simulink model "ScpAp_VechilestateEstimation_L2p"  (R2025b)
settings: Solver=FixedStepDiscrete  StartTime=0.0  StopTime=10.0  FixedStep=0.01  RelTol=1e-3
model workspace (MAT data in the model file):
  Accel_Diff_Th = Simulink.Parameter
  Accel_Diff_Th.Value = 1
  Accel_Diff_Th.Complexity = 'real'
  Accel_Diff_Th.Dimensions = [1 1]
  Accel_Diff_Th.DataType = 'auto'
  DT = Simulink.Parameter
  DT.Value = 0.01
  DT.Complexity = 'real'
  DT.Dimensions = [1 1]
  DT.DataType = 'auto'
  Speed_Diff_Th = Simulink.Parameter
  Speed_Diff_Th.Value = 4
  Speed_Diff_Th.Complexity = 'real'
  Speed_Diff_Th.Dimensions = [1 1]
  Speed_Diff_Th.DataType = 'auto'
  W1 = Simulink.Parameter
  W1.Value = 0.3
  W1.Complexity = 'real'
  W1.Dimensions = [1 1]
  W1.DataType = 'auto'
  W2 = Simulink.Parameter
  W2.Value = 0.7
  W2.Complexity = 'real'
  W2.Dimensions = [1 1]
  W2.DataType = 'auto'
  Wheel_Diff_Th = Simulink.Parameter
  Wheel_Diff_Th.Value = 5
  Wheel_Diff_Th.Complexity = 'real'
  Wheel_Diff_Th.Dimensions = [1 1]
  Wheel_Diff_Th.DataType = 'auto'
undefined symbols (not defined in the file): w_accel1, w_accel2, WhlSpd_Max, WhlSpd_Min
settings Model: DataDictionary=EgasPOC.sldd  Creator=IAST283  LastModifiedBy=IAST283
settings DataIOCC: SaveFormat=StructureWithTime
settings OptimizationCC: DefaultParameterBehavior=Inlined  EnhancedBackFolding=on  PassReuseOutputArgsAs=Individual arguments  ZeroExternalMemoryAtStartup=off  ZeroInternalMemoryAtStartup=off  OptimizeBlockOrder=speed  DifferentSizesBufferReuse=on  OptimizationCustomize=off  EfficientTunableParamExpr=on
settings DebuggingCC: ParameterTunabilityLossMsg=error
settings SFSimCC: MATLABDynamicMemAlloc=off
settings RTWCC: SystemTargetFile=autosar.tlc  GenCodeOnly=on  TemplateMakefile=ert_default_tmf  DataTypeReplacement=CDataTypesFixedWidth  Description=AUTOSAR
settings CodeAppCC: ForceParamTrailComments=on  IgnoreCustomStorageClasses=off  OperatorAnnotations=on  SimulinkDataObjDesc=on  SFDataObjDesc=on  InsertBlockDesc=on
settings STFCustomTargetCC: SystemTargetFile=autosar.tlc  TargetLangStandard=C99 (ISO)  MultiwordLength=256.0  ParMdlRefBuildCompliant=on  CompOptLevelCompliant=on  ConcurrentExecutionCompliant=off  IncludeMdlTerminateFcn=off  CombineOutputUpdateFcns=on  SuppressErrorStatus=on  ERTCustomFileBanners=on  SupportNonFinite=off  SupportComplex=off  SupportContinuousTime=off  SupportNonInlinedSFcns=off  RemoveResetFunc=on  MATLABClassNameForMDSCustomization=Simulink.SoftwareTarget.ERTCustomization  AutosarCompliant=on  GRTInterface=off  UseToolchainInfoCompliant=on  LookupTableObjectStructAxisOrder=2,1,3,4,...  LUTObjectStructOrderEvenSpacing=Size,Table,Breakpoints  AutosarCompilerAbstraction=off  DisableAUTOSARRoutinesHostLibrary=off  AutosarSchemaVersion=R23-11  AutosarMaxShortNameLength=128.0  AutosarMatrixIOAsArray=off
settings ERTTargetCC: ERTCustomFileTemplate=example_file_process.tlc  BooleanTrueId=TRUE  BooleanFalseId=FALSE  TargetLangStandard=C99 (ISO)  ConcurrentExecutionCompliant=off  IncludeMdlTerminateFcn=off  SuppressErrorStatus=on  SupportNonFinite=off  SupportComplex=off  ModelStepFunctionPrototypeControlCompliant=off  CPPClassGenCompliant=off  AutosarCompliant=on  LookupTableObjectStructAxisOrder=2,1,3,4,...  LUTObjectStructOrderEvenSpacing=Size,Table,Breakpoints

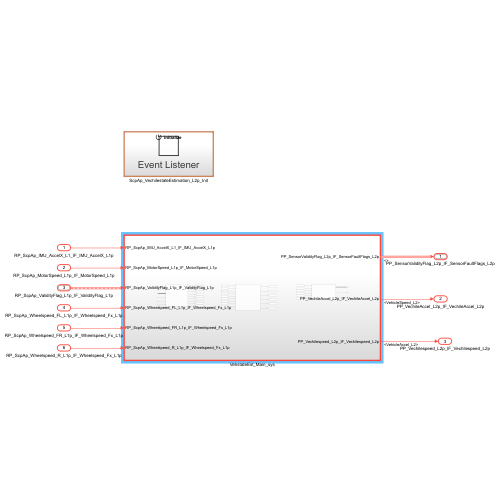
[thumbnail: Simulink's stored preview of the top-level diagram]
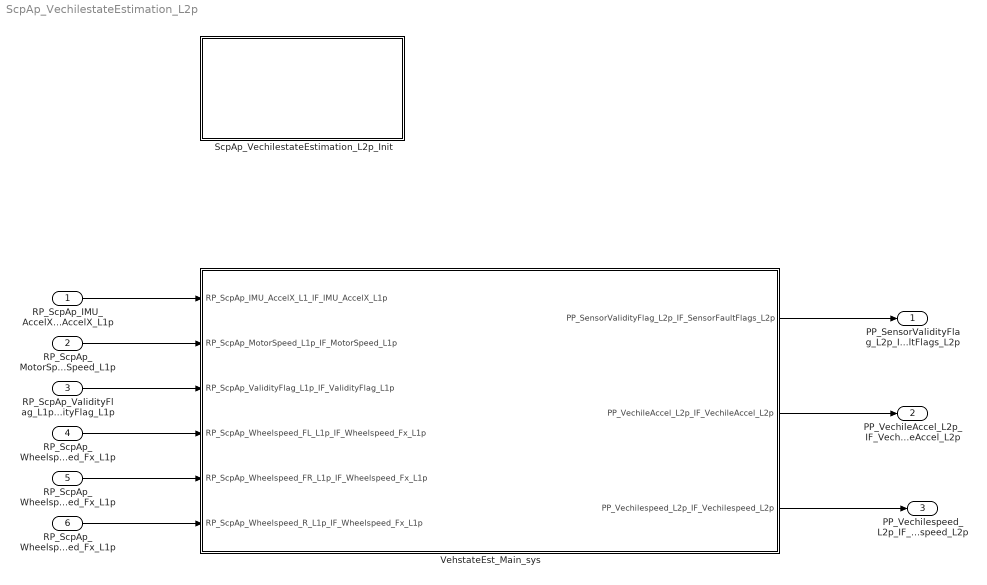
== system ScpAp_VechilestateEstimation_L2p ==
  RP_ScpAp_IMU_AccelX_L1_IF_IMU_AccelX_L1p : Inport  OutDataTypeStr=single  PortDimensions=1
  RP_ScpAp_MotorSpeed_L1p_IF_MotorSpeed_L1p : Inport  Port=2  OutDataTypeStr=uint8  PortDimensions=1
  RP_ScpAp_ValidityFlag_L1p_IF_ValidityFlag_L1p : Inport  Port=3  OutDataTypeStr=Bus: IF_ValidityFlag_L1p_IDT  PortDimensions=1  BusOutputAsStruct=on
  RP_ScpAp_Wheelspeed_FL_L1p_IF_Wheelspeed_Fx_L1p : Inport  Port=4  OutDataTypeStr=uint16  PortDimensions=1
  RP_ScpAp_Wheelspeed_FR_L1p_IF_Wheelspeed_Fx_L1p : Inport  Port=5  OutDataTypeStr=uint16  PortDimensions=1
  RP_ScpAp_Wheelspeed_R_L1p_IF_Wheelspeed_Fx_L1p : Inport  Port=6  OutDataTypeStr=uint16  PortDimensions=1
  ScpAp_VechilestateEstimation_L2p_Init : Subsystem
  VehstateEst_Main_sys : Subsystem  TreatAsAtomicUnit=on  SystemSampleTime=0.01
  PP_SensorValidityFlag_L2p_IF_SensorFaultFlags_L2p : Outport  OutDataTypeStr=Bus: IF_SensorFaultFlgs_L2p_IDT  PortDimensions=1  BusOutputAsStruct=on
  PP_VechileAccel_L2p_IF_VechileAccel_L2p : Outport  Port=2  OutDataTypeStr=int16  PortDimensions=1
  PP_Vechilespeed_L2p_IF_Vechilespeed_L2p : Outport  Port=3  OutDataTypeStr=uint16  PortDimensions=1
  wires:
  VehstateEst_Main_sys/1(PP_SensorValidityFlag_L2p_IF_SensorFaultFlags_L2p) -> PP_SensorValidityFlag_L2p_IF_SensorFaultFlags_L2p/1
  VehstateEst_Main_sys/2(PP_VechileAccel_L2p_IF_VechileAccel_L2p) -> PP_VechileAccel_L2p_IF_VechileAccel_L2p/1
  VehstateEst_Main_sys/3(PP_Vechilespeed_L2p_IF_Vechilespeed_L2p) -> PP_Vechilespeed_L2p_IF_Vechilespeed_L2p/1
  RP_ScpAp_IMU_AccelX_L1_IF_IMU_AccelX_L1p/1 -> VehstateEst_Main_sys/1(RP_ScpAp_IMU_AccelX_L1_IF_IMU_AccelX_L1p)
  RP_ScpAp_MotorSpeed_L1p_IF_MotorSpeed_L1p/1 -> VehstateEst_Main_sys/2(RP_ScpAp_MotorSpeed_L1p_IF_MotorSpeed_L1p)
  RP_ScpAp_ValidityFlag_L1p_IF_ValidityFlag_L1p/1 -> VehstateEst_Main_sys/3(RP_ScpAp_ValidityFlag_L1p_IF_ValidityFlag_L1p)
  RP_ScpAp_Wheelspeed_FL_L1p_IF_Wheelspeed_Fx_L1p/1 -> VehstateEst_Main_sys/4(RP_ScpAp_Wheelspeed_FL_L1p_IF_Wheelspeed_Fx_L1p)
  RP_ScpAp_Wheelspeed_FR_L1p_IF_Wheelspeed_Fx_L1p/1 -> VehstateEst_Main_sys/5(RP_ScpAp_Wheelspeed_FR_L1p_IF_Wheelspeed_Fx_L1p)
  RP_ScpAp_Wheelspeed_R_L1p_IF_Wheelspeed_Fx_L1p/1 -> VehstateEst_Main_sys/6(RP_ScpAp_Wheelspeed_R_L1p_IF_Wheelspeed_Fx_L1p)

== system ScpAp_VechilestateEstimation_L2p/ScpAp_VechilestateEstimation_L2p_Init ==
  Event Listener : EventListener  EventName=reset

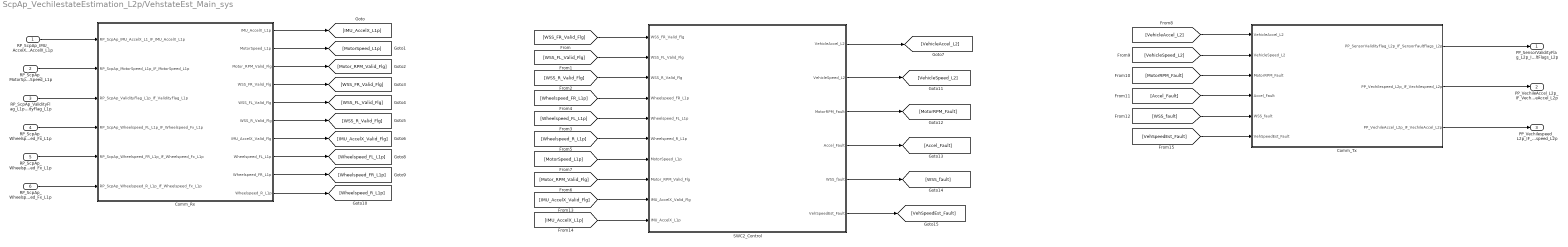
== system ScpAp_VechilestateEstimation_L2p/VehstateEst_Main_sys ==
  RP_ScpAp_IMU_AccelX_L1_IF_IMU_AccelX_L1p : Inport  OutDataTypeStr=single  PortDimensions=1
  RP_ScpAp_MotorSpeed_L1p_IF_MotorSpeed_L1p : Inport  Port=2  OutDataTypeStr=uint8  PortDimensions=1
  RP_ScpAp_ValidityFlag_L1p_IF_ValidityFlag_L1p : Inport  Port=3  OutDataTypeStr=Bus: IF_ValidityFlag_L1p_IDT  PortDimensions=1  BusOutputAsStruct=on
  RP_ScpAp_Wheelspeed_FL_L1p_IF_Wheelspeed_Fx_L1p : Inport  Port=4  OutDataTypeStr=uint16  PortDimensions=1
  RP_ScpAp_Wheelspeed_FR_L1p_IF_Wheelspeed_Fx_L1p : Inport  Port=5  OutDataTypeStr=uint16  PortDimensions=1
  RP_ScpAp_Wheelspeed_R_L1p_IF_Wheelspeed_Fx_L1p : Inport  Port=6  OutDataTypeStr=uint16  PortDimensions=1
  Comm_Rx : Subsystem
  Comm_Tx : Subsystem
  SWC2_Control : Subsystem  TreatAsAtomicUnit=on
  PP_SensorValidityFlag_L2p_IF_SensorFaultFlags_L2p : Outport
  PP_VechileAccel_L2p_IF_VechileAccel_L2p : Outport  Port=2
  PP_Vechilespeed_L2p_IF_Vechilespeed_L2p : Outport  Port=3
  wires:
  Comm_Rx/4(WSS_FR_Valid_Flg) -> [WSS_FR_Valid_Flg]
  Comm_Rx/3(Motor_RPM_Valid_Flg) -> [Motor_RPM_Valid_Flg]
  Comm_Rx/2(MotorSpeed_L1p) -> [MotorSpeed_L1p]
  Comm_Rx/8(Wheelspeed_FL_L1p) -> [Wheelspeed_FL_L1p]
  Comm_Rx/10(Wheelspeed_R_L1p) -> [Wheelspeed_R_L1p]
  Comm_Rx/9(Wheelspeed_FR_L1p) -> [Wheelspeed_FR_L1p]
  Comm_Rx/1(IMU_AccelX_L1p) -> [IMU_AccelX_L1p]
  Comm_Rx/7(IMU_AccelX_Valid_Flg) -> [IMU_AccelX_Valid_Flg]
  Comm_Rx/5(WSS_FL_Valid_Flg) -> [WSS_FL_Valid_Flg]
  Comm_Rx/6(WSS_R_Valid_Flg) -> [WSS_R_Valid_Flg]
  RP_ScpAp_IMU_AccelX_L1_IF_IMU_AccelX_L1p/1 -> Comm_Rx/1(RP_ScpAp_IMU_AccelX_L1_IF_IMU_AccelX_L1p)
  RP_ScpAp_MotorSpeed_L1p_IF_MotorSpeed_L1p/1 -> Comm_Rx/2(RP_ScpAp_MotorSpeed_L1p_IF_MotorSpeed_L1p)
  SWC2_Control/1("VehicleAccel_L2 ") -> [VehicleAccel_L2]
  SWC2_Control/3("MotorRPM_Fault ") -> [MotorRPM_Fault]
  [Wheelspeed_R_L1p] -> SWC2_Control/6(Wheelspeed_R_L1p)
  [IMU_AccelX_L1p] -> SWC2_Control/10(IMU_AccelX_L1p)
  SWC2_Control/6(VehSpeedEst_Fault) -> [VehSpeedEst_Fault]
  [MotorSpeed_L1p] -> SWC2_Control/7(MotorSpeed_L1p)
  [WSS_R_Valid_Flg] -> SWC2_Control/3(WSS_R_Valid_Flg)
  [IMU_AccelX_Valid_Flg] -> SWC2_Control/9(IMU_AccelX_Valid_Flg)
  [Wheelspeed_FR_L1p] -> SWC2_Control/4(Wheelspeed_FR_L1p)
  [Motor_RPM_Valid_Flg] -> SWC2_Control/8(Motor_RPM_Valid_Flg)
  [WSS_FR_Valid_Flg] -> SWC2_Control/1(WSS_FR_Valid_Flg)
  SWC2_Control/4(Accel_Fault) -> [Accel_Fault]
  [Wheelspeed_FL_L1p] -> SWC2_Control/5(Wheelspeed_FL_L1p)
  SWC2_Control/2("VehicleSpeed_L2 ") -> [VehicleSpeed_L2]
  [WSS_FL_Valid_Flg] -> SWC2_Control/2(WSS_FL_Valid_Flg)
  SWC2_Control/5("WSS_fault ") -> [WSS_fault]
  [VehicleAccel_L2] -> Comm_Tx/1(VehicleAccel_L2)
  [Accel_Fault] -> Comm_Tx/4(Accel_Fault)
  [MotorRPM_Fault] -> Comm_Tx/3(MotorRPM_Fault)
  [VehSpeedEst_Fault] -> Comm_Tx/6(VehSpeedEst_Fault)
  [WSS_fault] -> Comm_Tx/5(WSS_fault)
  [VehicleSpeed_L2] -> Comm_Tx/2(VehicleSpeed_L2)
  Comm_Tx/3(PP_VechileAccel_L2p_IF_VechileAccel_L2p) -> PP_Vechilespeed_L2p_IF_Vechilespeed_L2p/1
  Comm_Tx/1(PP_SensorValidityFlag_L2p_IF_SensorFaultFlags_L2p) -> PP_SensorValidityFlag_L2p_IF_SensorFaultFlags_L2p/1
  Comm_Tx/2(PP_Vechilespeed_L2p_IF_Vechilespeed_L2p) -> PP_VechileAccel_L2p_IF_VechileAccel_L2p/1
  RP_ScpAp_ValidityFlag_L1p_IF_ValidityFlag_L1p/1 -> Comm_Rx/3(RP_ScpAp_ValidityFlag_L1p_IF_ValidityFlag_L1p)
  RP_ScpAp_Wheelspeed_R_L1p_IF_Wheelspeed_Fx_L1p/1 -> Comm_Rx/6(RP_ScpAp_Wheelspeed_R_L1p_IF_Wheelspeed_Fx_L1p)
  RP_ScpAp_Wheelspeed_FR_L1p_IF_Wheelspeed_Fx_L1p/1 -> Comm_Rx/5(RP_ScpAp_Wheelspeed_FR_L1p_IF_Wheelspeed_Fx_L1p)
  RP_ScpAp_Wheelspeed_FL_L1p_IF_Wheelspeed_Fx_L1p/1 -> Comm_Rx/4(RP_ScpAp_Wheelspeed_FL_L1p_IF_Wheelspeed_Fx_L1p)

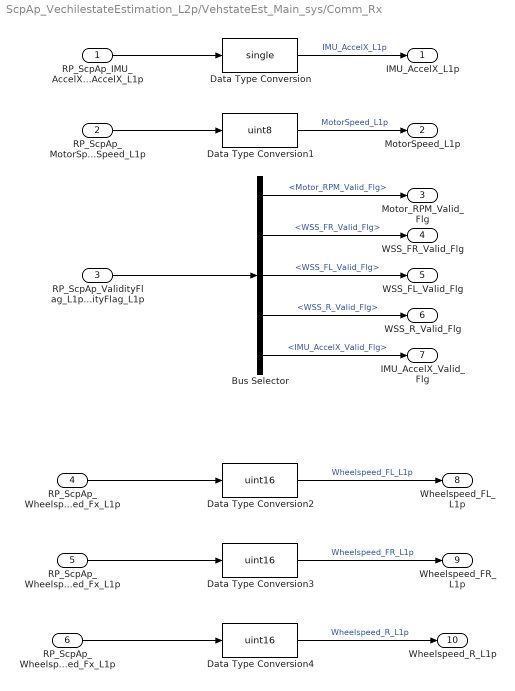
== system ScpAp_VechilestateEstimation_L2p/VehstateEst_Main_sys/Comm_Rx ==
  RP_ScpAp_IMU_AccelX_L1_IF_IMU_AccelX_L1p : Inport  OutDataTypeStr=single
  RP_ScpAp_MotorSpeed_L1p_IF_MotorSpeed_L1p : Inport  Port=2
  RP_ScpAp_ValidityFlag_L1p_IF_ValidityFlag_L1p : Inport  Port=3
  RP_ScpAp_Wheelspeed_FL_L1p_IF_Wheelspeed_Fx_L1p : Inport  Port=4
  RP_ScpAp_Wheelspeed_FR_L1p_IF_Wheelspeed_Fx_L1p : Inport  Port=5
  RP_ScpAp_Wheelspeed_R_L1p_IF_Wheelspeed_Fx_L1p : Inport  Port=6
  Bus Selector : BusSelector  OutputSignals=Motor_RPM_Valid_Flg,WSS_FR_Valid_Flg,WSS_FL_Valid_Flg,WSS_R_Valid_Flg,IMU_AccelX_Valid_Flg
  Data Type Conversion : DataTypeConversion  OutDataTypeStr=single  SaturateOnIntegerOverflow=off  RndMeth=Floor
  Data Type Conversion1 : DataTypeConversion  OutDataTypeStr=uint8  SaturateOnIntegerOverflow=off  RndMeth=Floor
  Data Type Conversion2 : DataTypeConversion  OutDataTypeStr=uint16  SaturateOnIntegerOverflow=off  RndMeth=Floor
  Data Type Conversion3 : DataTypeConversion  OutDataTypeStr=uint16  SaturateOnIntegerOverflow=off  RndMeth=Floor
  Data Type Conversion4 : DataTypeConversion  OutDataTypeStr=uint16  SaturateOnIntegerOverflow=off  RndMeth=Floor
  IMU_AccelX_L1p : Outport  OutDataTypeStr=single
  MotorSpeed_L1p : Outport  Port=2
  Motor_RPM_Valid_Flg : Outport  Port=3
  WSS_FR_Valid_Flg : Outport  Port=4
  WSS_FL_Valid_Flg : Outport  Port=5
  WSS_R_Valid_Flg : Outport  Port=6
  IMU_AccelX_Valid_Flg : Outport  Port=7
  Wheelspeed_FL_L1p : Outport  Port=8
  Wheelspeed_FR_L1p : Outport  Port=9
  Wheelspeed_R_L1p : Outport  Port=10
  wires:
  RP_ScpAp_IMU_AccelX_L1_IF_IMU_AccelX_L1p/1 -> Data Type Conversion/1
  RP_ScpAp_MotorSpeed_L1p_IF_MotorSpeed_L1p/1 -> Data Type Conversion1/1
  RP_ScpAp_ValidityFlag_L1p_IF_ValidityFlag_L1p/1 -> Bus Selector/1
  Bus Selector/1 -> Motor_RPM_Valid_Flg/1  "<Motor_RPM_Valid_Flg>"
  Bus Selector/2 -> WSS_FR_Valid_Flg/1  "<WSS_FR_Valid_Flg>"
  Bus Selector/3 -> WSS_FL_Valid_Flg/1  "<WSS_FL_Valid_Flg>"
  Bus Selector/4 -> WSS_R_Valid_Flg/1  "<WSS_R_Valid_Flg>"
  Bus Selector/5 -> IMU_AccelX_Valid_Flg/1  "<IMU_AccelX_Valid_Flg>"
  RP_ScpAp_Wheelspeed_FL_L1p_IF_Wheelspeed_Fx_L1p/1 -> Data Type Conversion2/1
  RP_ScpAp_Wheelspeed_FR_L1p_IF_Wheelspeed_Fx_L1p/1 -> Data Type Conversion3/1
  RP_ScpAp_Wheelspeed_R_L1p_IF_Wheelspeed_Fx_L1p/1 -> Data Type Conversion4/1
  Data Type Conversion/1 -> IMU_AccelX_L1p/1  "IMU_AccelX_L1p"
  Data Type Conversion1/1 -> MotorSpeed_L1p/1  "MotorSpeed_L1p"
  Data Type Conversion2/1 -> Wheelspeed_FL_L1p/1  "Wheelspeed_FL_L1p"
  Data Type Conversion3/1 -> Wheelspeed_FR_L1p/1  "Wheelspeed_FR_L1p"
  Data Type Conversion4/1 -> Wheelspeed_R_L1p/1  "Wheelspeed_R_L1p"

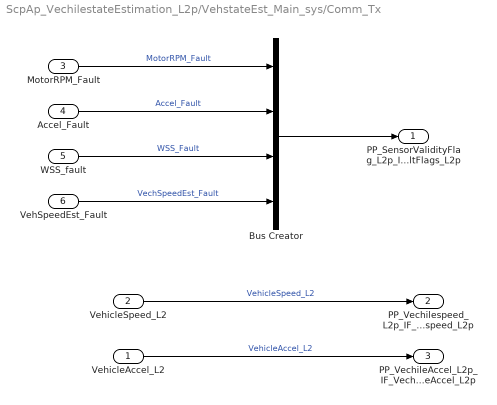
== system ScpAp_VechilestateEstimation_L2p/VehstateEst_Main_sys/Comm_Tx ==
  VehicleAccel_L2 : Inport
  VehicleSpeed_L2 : Inport  Port=2
  MotorRPM_Fault : Inport  Port=3
  Accel_Fault : Inport  Port=4
  WSS_fault : Inport  Port=5
  VehSpeedEst_Fault : Inport  Port=6
  Bus Creator : BusCreator  Inputs=4
  PP_SensorValidityFlag_L2p_IF_SensorFaultFlags_L2p : Outport
  PP_Vechilespeed_L2p_IF_Vechilespeed_L2p : Outport  Port=2
  PP_VechileAccel_L2p_IF_VechileAccel_L2p : Outport  Port=3
  wires:
  MotorRPM_Fault/1 -> Bus Creator/1  "MotorRPM_Fault"
  WSS_fault/1 -> Bus Creator/3  "WSS_Fault"
  Accel_Fault/1 -> Bus Creator/2  "Accel_Fault"
  VehSpeedEst_Fault/1 -> Bus Creator/4  "VechSpeedEst_Fault"
  VehicleAccel_L2/1 -> PP_VechileAccel_L2p_IF_VechileAccel_L2p/1  "VehicleAccel_L2"
  VehicleSpeed_L2/1 -> PP_Vechilespeed_L2p_IF_Vechilespeed_L2p/1  "VehicleSpeed_L2"
  Bus Creator/1 -> PP_SensorValidityFlag_L2p_IF_SensorFaultFlags_L2p/1

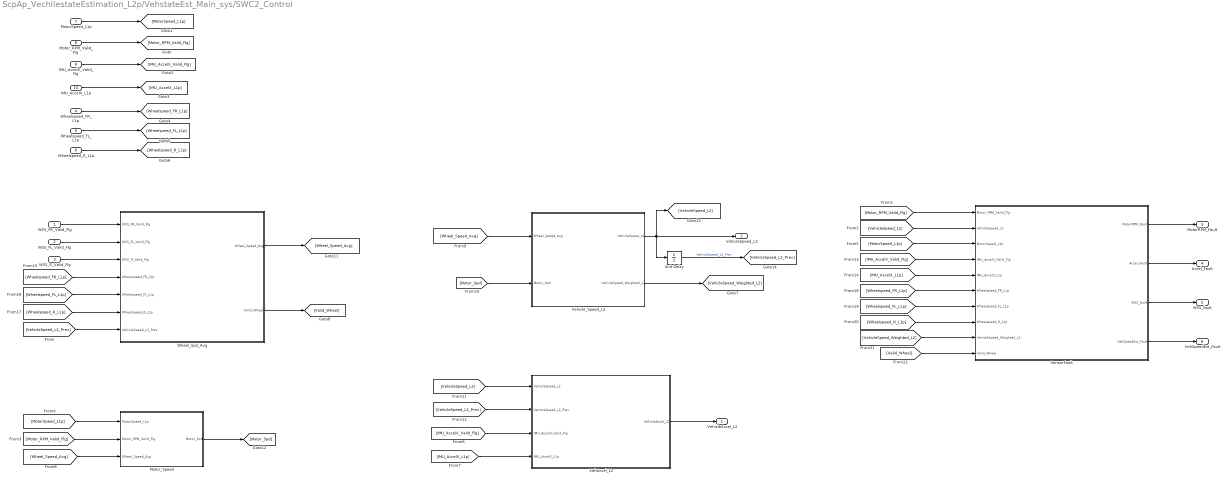
== system ScpAp_VechilestateEstimation_L2p/VehstateEst_Main_sys/SWC2_Control ==
  WSS_FR_Valid_Flg : Inport
  WSS_FL_Valid_Flg : Inport  Port=2
  WSS_R_Valid_Flg : Inport  Port=3
  Wheelspeed_FR_L1p : Inport  Port=4
  Wheelspeed_FL_L1p : Inport  Port=5
  Wheelspeed_R_L1p : Inport  Port=6
  MotorSpeed_L1p : Inport  Port=7
  Motor_RPM_Valid_Flg : Inport  Port=8
  IMU_AccelX_Valid_Flg : Inport  Port=9
  IMU_AccelX_L1p : Inport  Port=10
  Motor_Speed : Subsystem  TreatAsAtomicUnit=on
  SensorFault : Subsystem  TreatAsAtomicUnit=on
  Unit Delay : UnitDelay  SampleTime=-1  HasFrameUpgradeWarning=on
  VehAccel_L2 : Subsystem  TreatAsAtomicUnit=on
  Vehicle_Speed_L2 : Subsystem  TreatAsAtomicUnit=on
  Wheel_Spd_Avg : Subsystem  TreatAsAtomicUnit=on
  "VehicleAccel_L2 " : Outport
  "VehicleSpeed_L2 " : Outport  Port=2
  "MotorRPM_Fault " : Outport  Port=3
  Accel_Fault : Outport  Port=4
  "WSS_fault " : Outport  Port=5
  VehSpeedEst_Fault : Outport  Port=6
  wires:
  [Motor_Spd] -> Vehicle_Speed_L2/2(Motor_Spd)
  Motor_Speed/1(Motor_Spd) -> [Motor_Spd]
  Wheel_Spd_Avg/1(Wheel_Speed_Avg) -> [Wheel_Speed_Avg]
  [Wheel_Speed_Avg] -> Motor_Speed/3(Wheel_Speed_Avg)
  [Wheel_Speed_Avg] -> Vehicle_Speed_L2/1(Wheel_Speed_Avg)
  Unit Delay/1 -> [VehicleSpeed_L2_Prev]  "VehicleSpeed_L2_Prev"
  [VehicleSpeed_L2] -> VehAccel_L2/1(VehicleSpeed_L2)
  [VehicleSpeed_L2_Prev] -> VehAccel_L2/2(VehicleSpeed_L2_Prev)
  WSS_FR_Valid_Flg/1 -> Wheel_Spd_Avg/1(WSS_FR_Valid_Flg)
  WSS_R_Valid_Flg/1 -> Wheel_Spd_Avg/3(WSS_R_Valid_Flg)
  WSS_FL_Valid_Flg/1 -> Wheel_Spd_Avg/2(WSS_FL_Valid_Flg)
  VehAccel_L2/1("VehicleAccel_L2 ") -> "VehicleAccel_L2 "/1
  [VehicleSpeed_L2_Prev] -> Wheel_Spd_Avg/7(VehicleSpeed_L2_Prev)
  Motor_RPM_Valid_Flg/1 -> [Motor_RPM_Valid_Flg]
  [Motor_RPM_Valid_Flg] -> Motor_Speed/2(Motor_RPM_Valid_Flg)
  [MotorSpeed_L1p] -> Motor_Speed/1(MotorSpeed_L1p)
  [Motor_RPM_Valid_Flg] -> SensorFault/1(Motor_RPM_Valid_Flg)
  [VehicleSpeed_L2] -> SensorFault/2(VehicleSpeed_L2)
  [MotorSpeed_L1p] -> SensorFault/3(MotorSpeed_L1p)
  IMU_AccelX_Valid_Flg/1 -> [IMU_AccelX_Valid_Flg]
  IMU_AccelX_L1p/1 -> [IMU_AccelX_L1p]
  [IMU_AccelX_Valid_Flg] -> VehAccel_L2/3(IMU_AccelX_Valid_Flg)
  [IMU_AccelX_L1p] -> VehAccel_L2/4(IMU_AccelX_L1p)
  [IMU_AccelX_Valid_Flg] -> SensorFault/4(IMU_AccelX_Valid_Flg)
  [IMU_AccelX_L1p] -> SensorFault/5(IMU_AccelX_L1p)
  Wheelspeed_FR_L1p/1 -> [Wheelspeed_FR_L1p]
  Wheelspeed_FL_L1p/1 -> [Wheelspeed_FL_L1p]
  Wheelspeed_R_L1p/1 -> [Wheelspeed_R_L1p]
  [Wheelspeed_FR_L1p] -> Wheel_Spd_Avg/4(Wheelspeed_FR_L1p)
  [Wheelspeed_FL_L1p] -> Wheel_Spd_Avg/5(Wheelspeed_FL_L1p)
  [Wheelspeed_R_L1p] -> Wheel_Spd_Avg/6(Wheelspeed_R_L1p)
  [Wheelspeed_R_L1p] -> SensorFault/8(Wheelspeed_R_L1p)
  [Wheelspeed_FL_L1p] -> SensorFault/7(Wheelspeed_FL_L1p)
  [Wheelspeed_FR_L1p] -> SensorFault/6(Wheelspeed_FR_L1p)
  Vehicle_Speed_L2/2(VehicleSpeed_Weighted_L2) -> [VehicleSpeed_Weighted_L2]
  [VehicleSpeed_Weighted_L2] -> SensorFault/9(VehicleSpeed_Weighted_L2)
  Vehicle_Speed_L2/1("VehicleSpeed_L2 ") -> Unit Delay/1, [VehicleSpeed_L2], "VehicleSpeed_L2 "/1
  Wheel_Spd_Avg/2(Valid_Wheel) -> [Valid_Wheel]
  [Valid_Wheel] -> SensorFault/10(Valid_Wheel)
  SensorFault/1("MotorRPM_Fault ") -> "MotorRPM_Fault "/1
  SensorFault/2(Accel_Fault) -> Accel_Fault/1
  SensorFault/4(VehSpeedEst_Fault) -> VehSpeedEst_Fault/1
  SensorFault/3("WSS_fault ") -> "WSS_fault "/1
  MotorSpeed_L1p/1 -> [MotorSpeed_L1p]

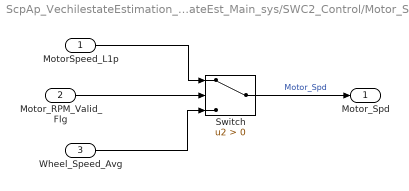
== system ScpAp_VechilestateEstimation_L2p/VehstateEst_Main_sys/SWC2_Control/Motor_Speed ==
  MotorSpeed_L1p : Inport
  Motor_RPM_Valid_Flg : Inport  Port=2
  Wheel_Speed_Avg : Inport  Port=3
  Switch : Switch  Criteria=u2 > Threshold  SaturateOnIntegerOverflow=off  InputSameDT=off
  Motor_Spd : Outport
  wires:
  Motor_RPM_Valid_Flg/1 -> Switch/2
  MotorSpeed_L1p/1 -> Switch/1
  Wheel_Speed_Avg/1 -> Switch/3
  Switch/1 -> Motor_Spd/1  "Motor_Spd"

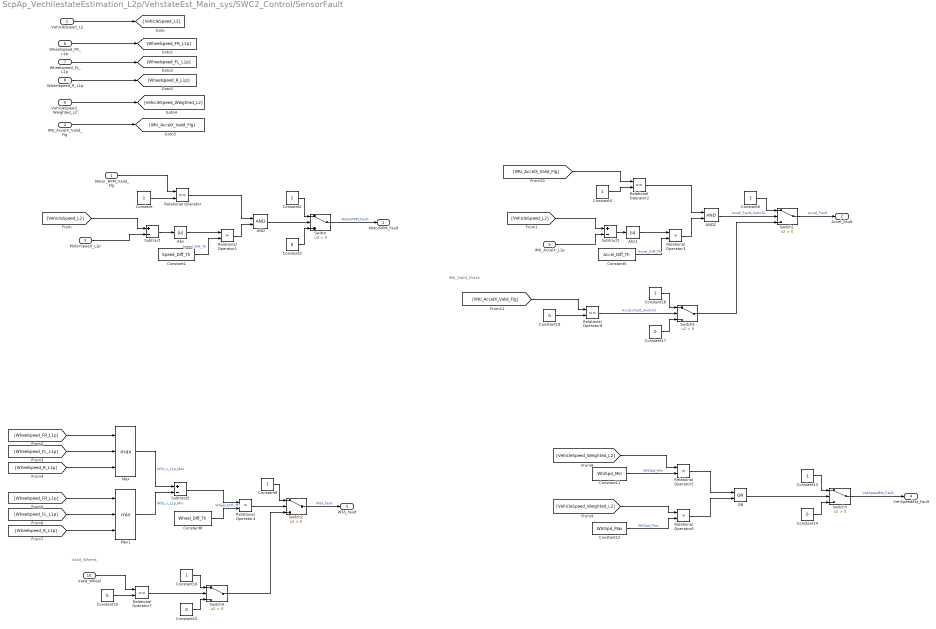
== system ScpAp_VechilestateEstimation_L2p/VehstateEst_Main_sys/SWC2_Control/SensorFault ==
  note: IMU_Valid_Ckeck
  note: Valid_Wheels
  Motor_RPM_Valid_Flg : Inport
  VehicleSpeed_L2 : Inport  Port=2
  MotorSpeed_L1p : Inport  Port=3
  IMU_AccelX_Valid_Flg : Inport  Port=4
  IMU_AccelX_L1p : Inport  Port=5  OutDataTypeStr=single
  Wheelspeed_FR_L1p : Inport  Port=6
  Wheelspeed_FL_L1p : Inport  Port=7
  Wheelspeed_R_L1p : Inport  Port=8
  VehicleSpeed_Weighted_L2 : Inport  Port=9
  Valid_Wheel : Inport  Port=10
  AND : Logic  AllPortsSameDT=off  OutDataTypeStr=boolean
  AND2 : Logic  AllPortsSameDT=off  OutDataTypeStr=boolean
  Abs : Abs  SaturateOnIntegerOverflow=off
  Abs1 : Abs  SaturateOnIntegerOverflow=off
  Constant : Constant
  Constant1 : Constant  Value=Speed_Diff_Th
  Constant10 : Constant  Value=0
  Constant11 : Constant  Value=WhlSpd_Min
  Constant12 : Constant  Value=WhlSpd_Max
  Constant{2,6,9,13,16,18} (6 alike) : Constant  OutDataTypeStr=boolean
  Constant{3,14..15,17} (4 alike) : Constant  Value=0  OutDataTypeStr=boolean
  Constant19 : Constant  Value=0
  Constant4 : Constant
  Constant5 : Constant  Value=Accel_Diff_Th
  Constant8 : Constant  Value=Wheel_Diff_Th
  Max : MinMax  Function=max  Inputs=3
  Max1 : MinMax  Inputs=3
  OR : Logic  Operator=OR  AllPortsSameDT=off  OutDataTypeStr=boolean
  Relational Operator{,2,7..8} (4 alike) : RelationalOperator  Operator===  OutDataTypeStr=boolean  RndMeth=Simplest  InputSameDT=off
  Relational Operator{1,3..4,6} (4 alike) : RelationalOperator  Operator=>  OutDataTypeStr=boolean  RndMeth=Simplest  InputSameDT=off
  Relational Operator5 : RelationalOperator  Operator=<  OutDataTypeStr=boolean  RndMeth=Simplest  InputSameDT=off
  Subtract : Sum  Inputs=+-
  Subtract1 : Sum  Inputs=+-
  Subtract2 : Sum  Inputs=+-
  Switch{,1..5} (6 alike) : Switch  Criteria=u2 > Threshold  SaturateOnIntegerOverflow=off  InputSameDT=off
  "MotorRPM_Fault " : Outport
  Accel_Fault : Outport  Port=2
  "WSS_fault " : Outport  Port=3
  VehSpeedEst_Fault : Outport  Port=4
  wires:
  Motor_RPM_Valid_Flg/1 -> Relational Operator/1
  Constant/1 -> Relational Operator/2
  MotorSpeed_L1p/1 -> Subtract/2
  Subtract/1 -> Abs/1
  Constant1/1 -> Relational Operator1/2  "Speed_Diff_Th"
  Switch/1 -> "MotorRPM_Fault "/1  "MotorRPM_Fault"
  Constant2/1 -> Switch/1
  Constant3/1 -> Switch/3
  VehicleSpeed_L2/1 -> [VehicleSpeed_L2]
  [VehicleSpeed_L2] -> Subtract/1
  Constant4/1 -> Relational Operator2/2
  [VehicleSpeed_L2] -> Subtract1/1
  IMU_AccelX_L1p/1 -> Subtract1/2
  Subtract1/1 -> Abs1/1
  Constant5/1 -> Relational Operator3/2  "Accel_Diff_Th"
  Constant6/1 -> Switch1/1
  Switch1/1 -> Accel_Fault/1  "Accel_Fault"
  Wheelspeed_FR_L1p/1 -> [Wheelspeed_FR_L1p]
  Wheelspeed_FL_L1p/1 -> [Wheelspeed_FL_L1p]
  Wheelspeed_R_L1p/1 -> [Wheelspeed_R_L1p]
  [Wheelspeed_FR_L1p] -> Max/1
  [Wheelspeed_FL_L1p] -> Max/2
  [Wheelspeed_R_L1p] -> Max/3
  Max/1 -> Subtract2/1  "WSS_x_L1p_Max"
  [Wheelspeed_FR_L1p] -> Max1/1
  [Wheelspeed_FL_L1p] -> Max1/2
  [Wheelspeed_R_L1p] -> Max1/3
  Max1/1 -> Subtract2/2  "WSS_x_L1p_Min"
  Subtract2/1 -> Relational Operator4/1
  Constant8/1 -> Relational Operator4/2  "Wheel_Diff_Th"
  Relational Operator4/1 -> Switch2/2
  Switch2/1 -> "WSS_fault "/1  "WSS_fault"
  Constant9/1 -> Switch2/1
  VehicleSpeed_Weighted_L2/1 -> [VehicleSpeed_Weighted_L2]
  [VehicleSpeed_Weighted_L2] -> Relational Operator5/1
  Constant11/1 -> Relational Operator5/2  "WhlSpd_Min"
  [VehicleSpeed_Weighted_L2] -> Relational Operator6/1
  Constant12/1 -> Relational Operator6/2  "WhlSpd_Max"
  Relational Operator5/1 -> OR/1
  Relational Operator6/1 -> OR/2
  OR/1 -> Switch3/2
  Switch3/1 -> VehSpeedEst_Fault/1  "VehSpeedEst_Fault"
  Constant13/1 -> Switch3/1
  Constant14/1 -> Switch3/3
  Valid_Wheel/1 -> Relational Operator7/1
  Constant10/1 -> Relational Operator7/2
  Relational Operator7/1 -> Switch4/2
  Constant16/1 -> Switch4/1
  Constant15/1 -> Switch4/3
  Switch4/1 -> Switch2/3
  IMU_AccelX_Valid_Flg/1 -> [IMU_AccelX_Valid_Flg]
  [IMU_AccelX_Valid_Flg] -> Relational Operator2/1
  [IMU_AccelX_Valid_Flg] -> Relational Operator8/1
  Constant19/1 -> Relational Operator8/2
  Relational Operator8/1 -> Switch5/2  "Accel_Fault_Switch2"
  Constant18/1 -> Switch5/1
  Constant17/1 -> Switch5/3
  Switch5/1 -> Switch1/3
  Abs/1 -> Relational Operator1/1
  Relational Operator/1 -> AND/1
  Relational Operator1/1 -> AND/2
  AND/1 -> Switch/2
  Relational Operator2/1 -> AND2/1
  Abs1/1 -> Relational Operator3/1
  Relational Operator3/1 -> AND2/2
  AND2/1 -> Switch1/2  "Accel_Fault_Switch1"

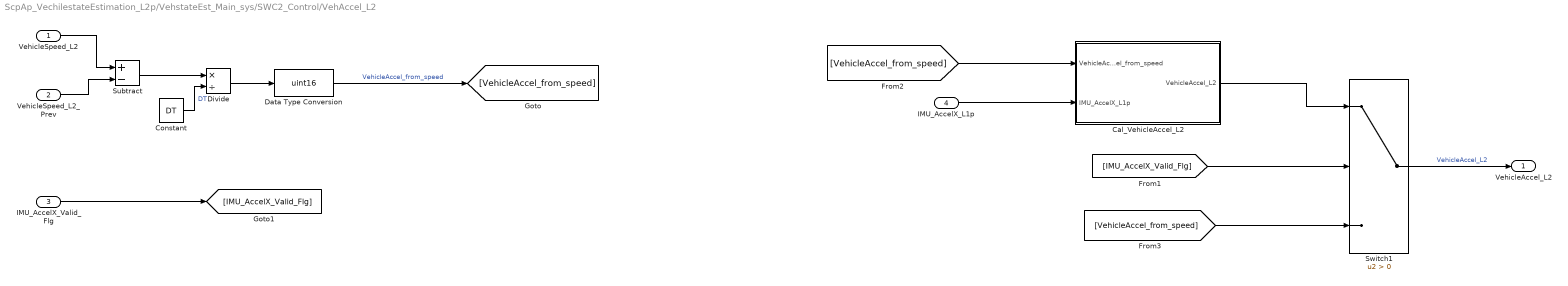
== system ScpAp_VechilestateEstimation_L2p/VehstateEst_Main_sys/SWC2_Control/VehAccel_L2 ==
  VehicleSpeed_L2 : Inport
  VehicleSpeed_L2_Prev : Inport  Port=2
  IMU_AccelX_Valid_Flg : Inport  Port=3
  IMU_AccelX_L1p : Inport  Port=4
  "Cal_VehicleAccel_L2 " : Subsystem  TreatAsAtomicUnit=on
  Constant : Constant  Value=DT
  Data Type Conversion : DataTypeConversion  OutDataTypeStr=uint16  SaturateOnIntegerOverflow=off  RndMeth=Floor
  Divide : Product  Inputs=*/
  Subtract : Sum  Inputs=+-
  Switch1 : Switch  Criteria=u2 > Threshold  SaturateOnIntegerOverflow=off  InputSameDT=off
  "VehicleAccel_L2 " : Outport
  wires:
  VehicleSpeed_L2/1 -> Subtract/1
  VehicleSpeed_L2_Prev/1 -> Subtract/2
  Subtract/1 -> Divide/1
  Constant/1 -> Divide/2  "DT"
  Divide/1 -> Data Type Conversion/1
  IMU_AccelX_Valid_Flg/1 -> [IMU_AccelX_Valid_Flg]
  [IMU_AccelX_Valid_Flg] -> Switch1/2
  Switch1/1 -> "VehicleAccel_L2 "/1  "VehicleAccel_L2"
  [VehicleAccel_from_speed] -> "Cal_VehicleAccel_L2 "/1(VehicleAccel_from_speed)
  IMU_AccelX_L1p/1 -> "Cal_VehicleAccel_L2 "/2(IMU_AccelX_L1p)
  "Cal_VehicleAccel_L2 "/1("VehicleAccel_L2 ") -> Switch1/1
  [VehicleAccel_from_speed] -> Switch1/3
  Data Type Conversion/1 -> [VehicleAccel_from_speed]  "VehicleAccel_from_speed"

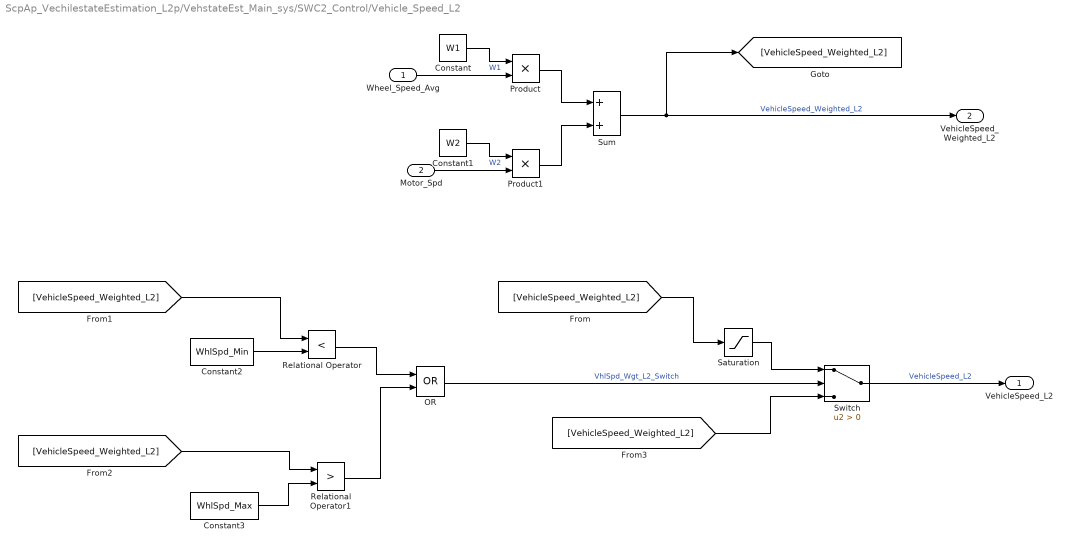
== system ScpAp_VechilestateEstimation_L2p/VehstateEst_Main_sys/SWC2_Control/Vehicle_Speed_L2 ==
  Wheel_Speed_Avg : Inport
  Motor_Spd : Inport  Port=2
  Constant : Constant  Value=W1  OutDataTypeStr=int16
  Constant1 : Constant  Value=W2  OutDataTypeStr=int16
  Constant2 : Constant  Value=WhlSpd_Min
  Constant3 : Constant  Value=WhlSpd_Max
  OR : Logic  Operator=OR  AllPortsSameDT=off  OutDataTypeStr=boolean
  Product : Product  OutDataTypeStr=int16
  Product1 : Product  OutDataTypeStr=int16
  Relational Operator : RelationalOperator  Operator=<  OutDataTypeStr=boolean  RndMeth=Simplest  InputSameDT=off
  Relational Operator1 : RelationalOperator  Operator=>  OutDataTypeStr=boolean  RndMeth=Simplest  InputSameDT=off
  Saturation : Saturate  UpperLimit=32  LowerLimit=0
  Sum : Sum
  Switch : Switch  Criteria=u2 > Threshold  SaturateOnIntegerOverflow=off  InputSameDT=off
  "VehicleSpeed_L2 " : Outport
  VehicleSpeed_Weighted_L2 : Outport  Port=2
  wires:
  Constant/1 -> Product/1  "W1"
  Wheel_Speed_Avg/1 -> Product/2
  Product/1 -> Sum/1
  Constant1/1 -> Product1/1  "W2"
  Motor_Spd/1 -> Product1/2
  Product1/1 -> Sum/2
  Sum/1 -> VehicleSpeed_Weighted_L2/1, [VehicleSpeed_Weighted_L2]  "VehicleSpeed_Weighted_L2"
  [VehicleSpeed_Weighted_L2] -> Saturation/1
  [VehicleSpeed_Weighted_L2] -> Relational Operator/1
  Constant2/1 -> Relational Operator/2
  Relational Operator/1 -> OR/1
  [VehicleSpeed_Weighted_L2] -> Relational Operator1/1
  Constant3/1 -> Relational Operator1/2
  Relational Operator1/1 -> OR/2
  OR/1 -> Switch/2  "VhlSpd_Wgt_L2_Switch"
  Switch/1 -> "VehicleSpeed_L2 "/1  "VehicleSpeed_L2"
  Saturation/1 -> Switch/1
  [VehicleSpeed_Weighted_L2] -> Switch/3

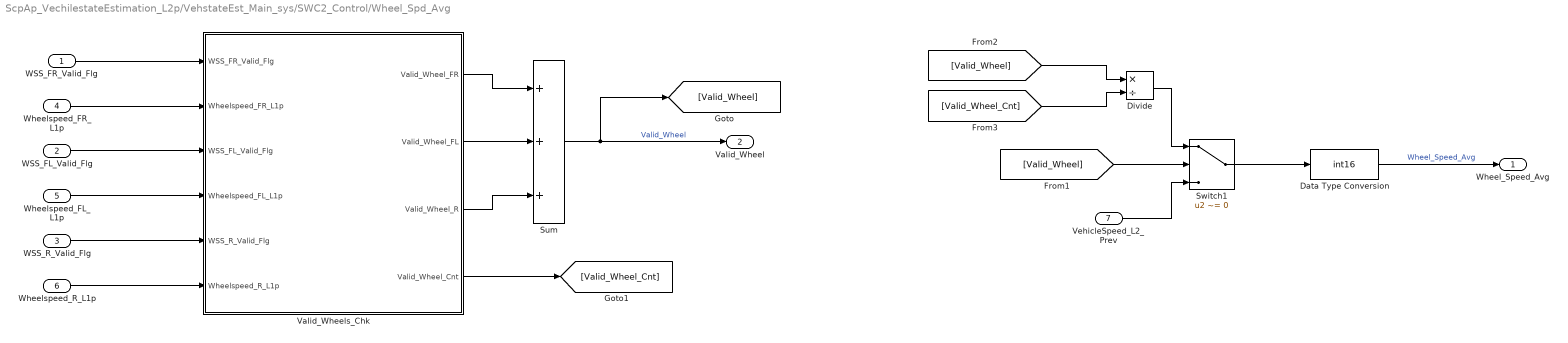
== system ScpAp_VechilestateEstimation_L2p/VehstateEst_Main_sys/SWC2_Control/Wheel_Spd_Avg ==
  WSS_FR_Valid_Flg : Inport
  WSS_FL_Valid_Flg : Inport  Port=2
  WSS_R_Valid_Flg : Inport  Port=3
  Wheelspeed_FR_L1p : Inport  Port=4
  Wheelspeed_FL_L1p : Inport  Port=5
  Wheelspeed_R_L1p : Inport  Port=6
  VehicleSpeed_L2_Prev : Inport  Port=7
  Data Type Conversion : DataTypeConversion  OutDataTypeStr=int16  SaturateOnIntegerOverflow=off  RndMeth=Floor
  Divide : Product  Inputs=*/
  Sum : Sum  Inputs=+++
  Switch1 : Switch  Criteria=u2 ~= 0  SaturateOnIntegerOverflow=off  InputSameDT=off
  Valid_Wheels_Chk : Subsystem  TreatAsAtomicUnit=on
  Wheel_Speed_Avg : Outport
  Valid_Wheel : Outport  Port=2
  wires:
  WSS_FR_Valid_Flg/1 -> Valid_Wheels_Chk/1(WSS_FR_Valid_Flg)
  Wheelspeed_FR_L1p/1 -> Valid_Wheels_Chk/2(Wheelspeed_FR_L1p)
  WSS_FL_Valid_Flg/1 -> Valid_Wheels_Chk/3(WSS_FL_Valid_Flg)
  Wheelspeed_FL_L1p/1 -> Valid_Wheels_Chk/4(Wheelspeed_FL_L1p)
  WSS_R_Valid_Flg/1 -> Valid_Wheels_Chk/5(WSS_R_Valid_Flg)
  Wheelspeed_R_L1p/1 -> Valid_Wheels_Chk/6(Wheelspeed_R_L1p)
  Valid_Wheels_Chk/1(Valid_Wheel_FR) -> Sum/1
  Valid_Wheels_Chk/2(Valid_Wheel_FL) -> Sum/2
  Valid_Wheels_Chk/3(Valid_Wheel_R) -> Sum/3
  Sum/1 -> Valid_Wheel/1, [Valid_Wheel]  "Valid_Wheel"
  Valid_Wheels_Chk/4(Valid_Wheel_Cnt) -> [Valid_Wheel_Cnt]
  Switch1/1 -> Data Type Conversion/1
  [Valid_Wheel] -> Switch1/2
  [Valid_Wheel] -> Divide/1
  [Valid_Wheel_Cnt] -> Divide/2
  Divide/1 -> Switch1/1
  VehicleSpeed_L2_Prev/1 -> Switch1/3
  Data Type Conversion/1 -> Wheel_Speed_Avg/1  "Wheel_Speed_Avg"

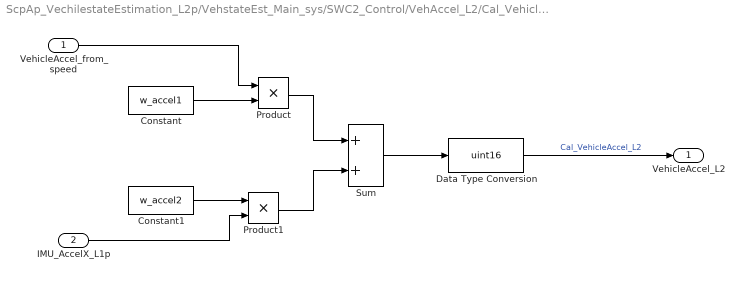
== system ScpAp_VechilestateEstimation_L2p/VehstateEst_Main_sys/SWC2_Control/VehAccel_L2/Cal_VehicleAccel_L2  ==
  VehicleAccel_from_speed : Inport
  IMU_AccelX_L1p : Inport  Port=2
  Constant : Constant  Value=w_accel1
  Constant1 : Constant  Value=w_accel2
  Data Type Conversion : DataTypeConversion  OutDataTypeStr=uint16  SaturateOnIntegerOverflow=off  RndMeth=Floor
  Product : Product
  Product1 : Product
  Sum : Sum
  "VehicleAccel_L2 " : Outport
  wires:
  Constant/1 -> Product/2
  VehicleAccel_from_speed/1 -> Product/1
  Product/1 -> Sum/1
  Constant1/1 -> Product1/1
  IMU_AccelX_L1p/1 -> Product1/2
  Product1/1 -> Sum/2
  Sum/1 -> Data Type Conversion/1
  Data Type Conversion/1 -> "VehicleAccel_L2 "/1  "Cal_VehicleAccel_L2"

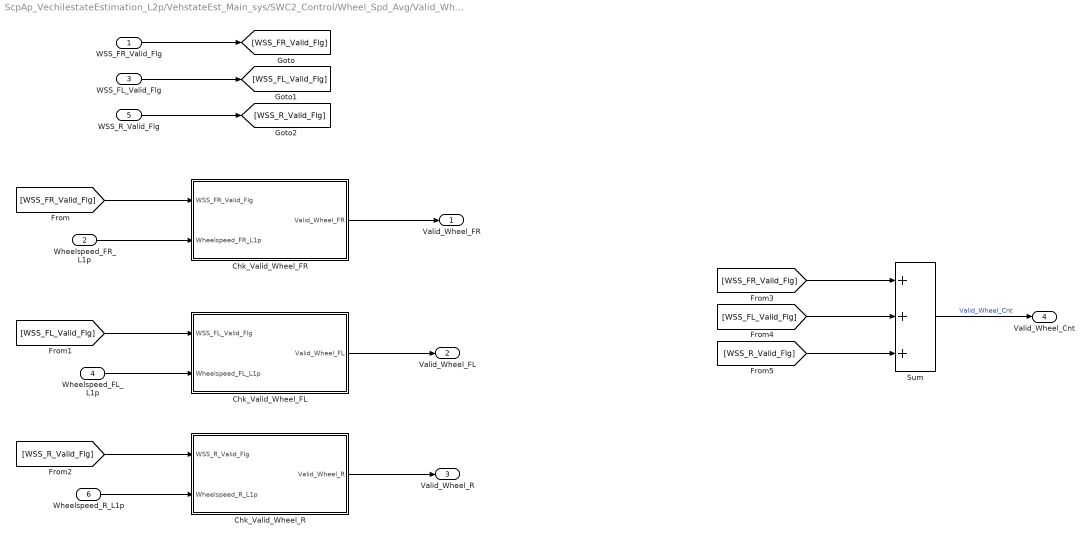
== system ScpAp_VechilestateEstimation_L2p/VehstateEst_Main_sys/SWC2_Control/Wheel_Spd_Avg/Valid_Wheels_Chk ==
  WSS_FR_Valid_Flg : Inport
  Wheelspeed_FR_L1p : Inport  Port=2
  WSS_FL_Valid_Flg : Inport  Port=3
  Wheelspeed_FL_L1p : Inport  Port=4
  WSS_R_Valid_Flg : Inport  Port=5
  Wheelspeed_R_L1p : Inport  Port=6
  Chk_Valid_Wheel_FL : Subsystem  TreatAsAtomicUnit=on
  Chk_Valid_Wheel_FR : Subsystem  TreatAsAtomicUnit=on
  Chk_Valid_Wheel_R : Subsystem  TreatAsAtomicUnit=on
  Sum : Sum  Inputs=+++
  Valid_Wheel_FR : Outport
  Valid_Wheel_FL : Outport  Port=2
  Valid_Wheel_R : Outport  Port=3
  Valid_Wheel_Cnt : Outport  Port=4
  wires:
  Chk_Valid_Wheel_FL/1(Valid_Wheel_FL) -> Valid_Wheel_FL/1
  Wheelspeed_FR_L1p/1 -> Chk_Valid_Wheel_FR/2(Wheelspeed_FR_L1p)
  Chk_Valid_Wheel_FR/1(Valid_Wheel_FR) -> Valid_Wheel_FR/1
  Wheelspeed_R_L1p/1 -> Chk_Valid_Wheel_R/2(Wheelspeed_R_L1p)
  Wheelspeed_FL_L1p/1 -> Chk_Valid_Wheel_FL/2(Wheelspeed_FL_L1p)
  Chk_Valid_Wheel_R/1(Valid_Wheel_R) -> Valid_Wheel_R/1
  WSS_FR_Valid_Flg/1 -> [WSS_FR_Valid_Flg]
  WSS_FL_Valid_Flg/1 -> [WSS_FL_Valid_Flg]
  WSS_R_Valid_Flg/1 -> [WSS_R_Valid_Flg]
  [WSS_FR_Valid_Flg] -> Chk_Valid_Wheel_FR/1(WSS_FR_Valid_Flg)
  [WSS_FL_Valid_Flg] -> Chk_Valid_Wheel_FL/1(WSS_FL_Valid_Flg)
  [WSS_R_Valid_Flg] -> Chk_Valid_Wheel_R/1(WSS_R_Valid_Flg)
  [WSS_FL_Valid_Flg] -> Sum/2
  [WSS_FR_Valid_Flg] -> Sum/1
  [WSS_R_Valid_Flg] -> Sum/3
  Sum/1 -> Valid_Wheel_Cnt/1  "Valid_Wheel_Cnt"

== system ScpAp_VechilestateEstimation_L2p/VehstateEst_Main_sys/SWC2_Control/Wheel_Spd_Avg/Valid_Wheels_Chk/Chk_Valid_Wheel_FL ==
  WSS_FL_Valid_Flg : Inport
  Wheelspeed_FL_L1p : Inport  Port=2
  Constant : Constant  Value=0
  Switch : Switch  Criteria=u2 > Threshold  SaturateOnIntegerOverflow=off  InputSameDT=off
  Valid_Wheel_FL : Outport
  wires:
  WSS_FL_Valid_Flg/1 -> Switch/2
  Wheelspeed_FL_L1p/1 -> Switch/1
  Constant/1 -> Switch/3
  Switch/1 -> Valid_Wheel_FL/1  "Valid_Wheel_FL"

== system ScpAp_VechilestateEstimation_L2p/VehstateEst_Main_sys/SWC2_Control/Wheel_Spd_Avg/Valid_Wheels_Chk/Chk_Valid_Wheel_FR ==
  WSS_FR_Valid_Flg : Inport
  Wheelspeed_FR_L1p : Inport  Port=2
  Constant : Constant  Value=0
  Switch : Switch  Criteria=u2 > Threshold  SaturateOnIntegerOverflow=off  InputSameDT=off
  Valid_Wheel_FR : Outport
  wires:
  WSS_FR_Valid_Flg/1 -> Switch/2
  Wheelspeed_FR_L1p/1 -> Switch/1
  Constant/1 -> Switch/3
  Switch/1 -> Valid_Wheel_FR/1  "Valid_Wheel_FR"

== system ScpAp_VechilestateEstimation_L2p/VehstateEst_Main_sys/SWC2_Control/Wheel_Spd_Avg/Valid_Wheels_Chk/Chk_Valid_Wheel_R ==
  WSS_R_Valid_Flg : Inport
  Wheelspeed_R_L1p : Inport  Port=2
  Constant : Constant  Value=0
  Switch : Switch  Criteria=u2 > Threshold  SaturateOnIntegerOverflow=off  InputSameDT=off
  Valid_Wheel_R : Outport
  wires:
  Switch/1 -> Valid_Wheel_R/1  "Valid_Wheel_R"
  Constant/1 -> Switch/3
  Wheelspeed_R_L1p/1 -> Switch/1
  WSS_R_Valid_Flg/1 -> Switch/2
